simulink model "Chart"  (R2022a)
settings: Solver=FixedStepDiscrete  StartTime=0.0  StopTime=inf  RelTol=1e-3
settings Model: DVExtractedSubsystem=Chart  Creator=attit  LastModifiedBy=attit
settings DebuggingCC: FrameProcessingCompatibilityMsg=none
settings RTWCC: TLCOptions=-aAlwaysIncludeCustomSrc=1
settings ConfigComp: DVMaxProcessTime=4000  DVModelCoverageObjectives=MCDC  DVTestSuiteOptimization=Auto  DVDetectOutOfBounds=on  DVModelReferenceHarness=on  DVHarnessSource=Signal Editor

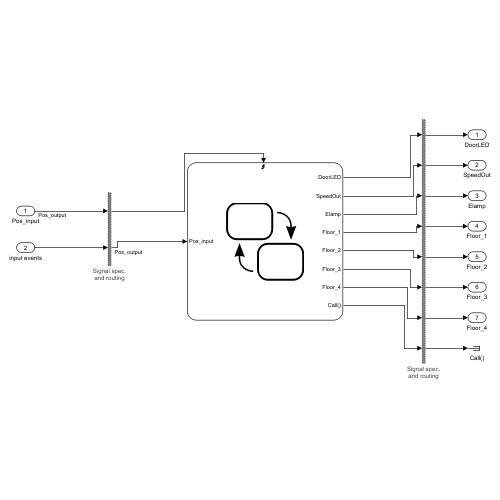
[thumbnail: Simulink's stored preview of the top-level diagram]
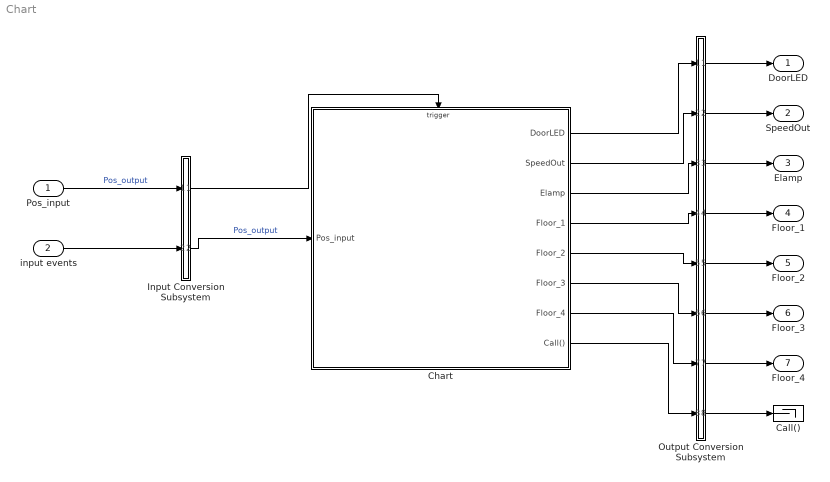
== system Chart ==
  Pos_input : Inport  OutDataTypeStr=double  PortDimensions=[1]  Interpolate=off
  input events : Inport  Port=2  OutDataTypeStr=double  PortDimensions=[7]  Interpolate=off
  Call() : Terminator
  Chart : Stateflow chart  TreatAsAtomicUnit=on
  Input Conversion Subsystem : Subsystem  Tag=__SLT_ICS__  Description=|
      | Signal spec.
      | and routing
      settings: AttributesFormatString=%<Description>
  Output Conversion Subsystem : Subsystem  Tag=__SLT_OCS__  Description=|
      | Signal spec.
      | and routing
      settings: AttributesFormatString=%<Description>
  DoorLED : Outport
  SpeedOut : Outport  Port=2
  Elamp : Outport  Port=3
  Floor_1 : Outport  Port=4
  Floor_2 : Outport  Port=5
  Floor_3 : Outport  Port=6
  Floor_4 : Outport  Port=7
  wires:
  Pos_input/1 -> Input Conversion Subsystem/1(Inport_1)  "Pos_output"
  input events/1 -> Input Conversion Subsystem/2(Inport_2)
  Output Conversion Subsystem/1(Outport_1) -> DoorLED/1
  Output Conversion Subsystem/2(Outport_2) -> SpeedOut/1
  Output Conversion Subsystem/3(Outport_3) -> Elamp/1
  Output Conversion Subsystem/4(Outport_4) -> Floor_1/1
  Output Conversion Subsystem/5(Outport_5) -> Floor_2/1
  Output Conversion Subsystem/6(Outport_6) -> Floor_3/1
  Output Conversion Subsystem/7(Outport_7) -> Floor_4/1
  Output Conversion Subsystem/8(Outport_8) -> Call()/1
  Input Conversion Subsystem/1(Outport_2) -> Chart/Trigger
  Input Conversion Subsystem/2(Outport_1) -> Chart/1(Pos_input)  "Pos_output"
  Chart/1(DoorLED) -> Output Conversion Subsystem/1(Inport_1)
  Chart/2(SpeedOut) -> Output Conversion Subsystem/2(Inport_2)
  Chart/3(Elamp) -> Output Conversion Subsystem/3(Inport_3)
  Chart/4(Floor_1) -> Output Conversion Subsystem/4(Inport_4)
  Chart/5(Floor_2) -> Output Conversion Subsystem/5(Inport_5)
  Chart/6(Floor_3) -> Output Conversion Subsystem/6(Inport_6)
  Chart/7(Floor_4) -> Output Conversion Subsystem/7(Inport_7)
  Chart/8(Call()) -> Output Conversion Subsystem/8(Inport_8)

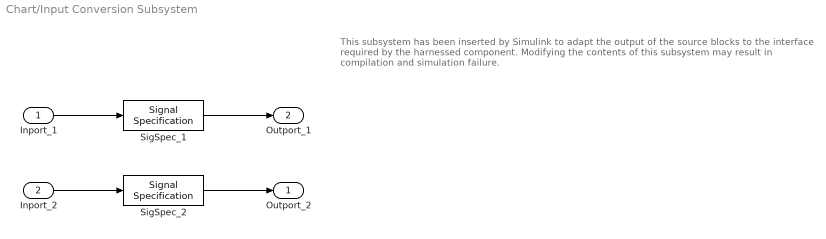
== system Chart/Input Conversion Subsystem ==
  note: This subsystem has been inserted by Simulink to adapt the output of the source blocks to the interface required by the harnessed component.
      |  Modifying the contents of this subsystem may result in compilation and simulation failure.
  Inport_1 : Inport
  Inport_2 : Inport  Port=2
  SigSpec_1 : SignalSpecification  OutDataTypeStr=double  Dimensions=[1]
  SigSpec_2 : SignalSpecification  OutDataTypeStr=double  Dimensions=[7]
  Outport_2 : Outport
  Outport_1 : Outport  Port=2
  wires:
  SigSpec_1/1 -> Outport_1/1
  Inport_1/1 -> SigSpec_1/1
  SigSpec_2/1 -> Outport_2/1
  Inport_2/1 -> SigSpec_2/1

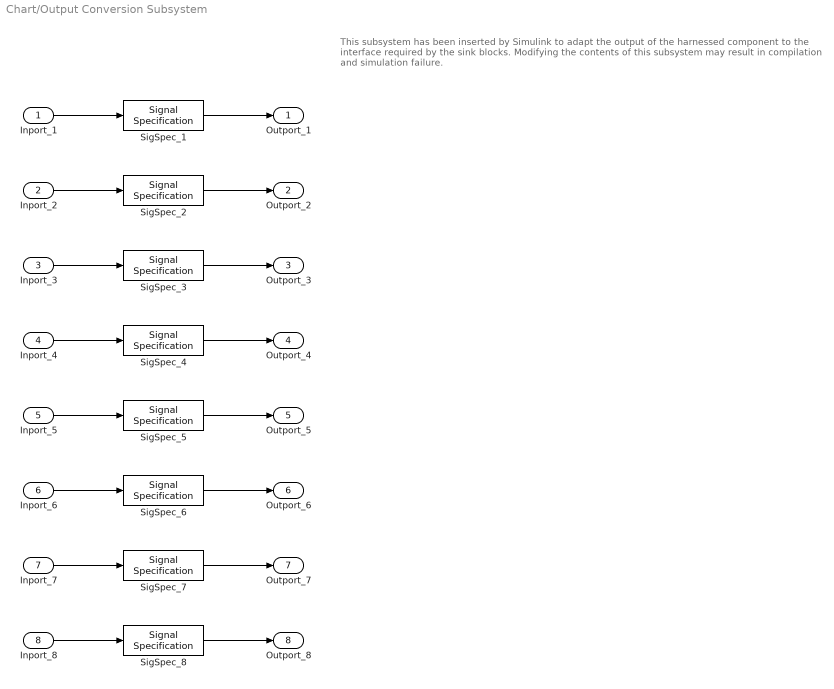
== system Chart/Output Conversion Subsystem ==
  note: This subsystem has been inserted by Simulink to adapt the output of the harnessed component to the interface required by the sink blocks.
      |  Modifying the contents of this subsystem may result in compilation and simulation failure.
  Inport_1 : Inport
  Inport_2 : Inport  Port=2
  Inport_3 : Inport  Port=3
  Inport_4 : Inport  Port=4
  Inport_5 : Inport  Port=5
  Inport_6 : Inport  Port=6
  Inport_7 : Inport  Port=7
  Inport_8 : Inport  Port=8
  SigSpec_{1..7} (7 alike) : SignalSpecification  OutDataTypeStr=double  Dimensions=[1]
  SigSpec_8 : SignalSpecification
  Outport_1 : Outport
  Outport_2 : Outport  Port=2
  Outport_3 : Outport  Port=3
  Outport_4 : Outport  Port=4
  Outport_5 : Outport  Port=5
  Outport_6 : Outport  Port=6
  Outport_7 : Outport  Port=7
  Outport_8 : Outport  Port=8
  wires:
  Inport_1/1 -> SigSpec_1/1
  SigSpec_1/1 -> Outport_1/1
  Inport_2/1 -> SigSpec_2/1
  SigSpec_2/1 -> Outport_2/1
  Inport_3/1 -> SigSpec_3/1
  SigSpec_3/1 -> Outport_3/1
  Inport_4/1 -> SigSpec_4/1
  SigSpec_4/1 -> Outport_4/1
  Inport_5/1 -> SigSpec_5/1
  SigSpec_5/1 -> Outport_5/1
  Inport_6/1 -> SigSpec_6/1
  SigSpec_6/1 -> Outport_6/1
  Inport_7/1 -> SigSpec_7/1
  SigSpec_7/1 -> Outport_7/1
  Inport_8/1 -> SigSpec_8/1
  SigSpec_8/1 -> Outport_8/1

== stateflow chart Chart/Chart ==
  state ElevatorUnitControl [parallel]
    settings: executionOrder=4
    state GO_DOWN
      entry:
      SpeedOut=-0.2
    state OFF
      entry:SpeedOut=0;
      Elamp=0;
    state GO_UP
      entry:SpeedOut=0.2
    state HALT
      entry:SpeedOut=0;
      Elamp=1
    (default) -> OFF
    OFF -> (junction 166) [order 1] : [in(LiftAlgorithm.MOTOR_ON)]
    (junction 166) -> GO_DOWN [order 1] : [Direction<Pos_input]
    GO_DOWN -> (junction 182) [order 1] : [Emergency]
    (junction 166) -> (junction 177) [order 2] : [Direction>Pos_input]
    (junction 182) -> (junction 183)
    GO_DOWN -> OFF [order 2] : [~in(LiftAlgorithm.MOTOR_ON)]
    GO_UP -> OFF [order 2] : [~in(LiftAlgorithm.MOTOR_ON)]
    HALT -> OFF : [Start]
    OFF -> HALT [order 2] : [Emergency]
    (junction 177) -> GO_UP
    GO_UP -> (junction 183) [order 1] : [Emergency]
    (junction 183) -> (junction 184)
    (junction 184) -> HALT
  state RequestServiced(pos) [function]
    note: Do not put any code along
        | the transitions that run
        | down the right side!
    (default) -> (junction 121)
    (junction 121) -> (junction 116) [order 1] : [pos == 1]
    (junction 121) -> (junction 131) [order 2]
    (junction 116) -> (junction 137) : {F1_press=0;}
    (junction 137) -> (junction 120)
    (junction 120) -> (junction 117)
    (junction 131) -> (junction 113) [order 1] : [pos == 2]
    (junction 131) -> (junction 123) [order 2]
    (junction 113) -> (junction 135) : {F2_press=0;}
    (junction 135) -> (junction 117)
    (junction 117) -> (junction 114)
    (junction 123) -> (junction 136) [order 1] : [pos == 3]
    (junction 123) -> (junction 122) [order 2]
    (junction 136) -> (junction 118) : {F3_press=0;}
    (junction 118) -> (junction 114)
    (junction 114) -> (junction 124)
    (junction 122) -> (junction 119) [order 1] : [pos == 4]
    (junction 122) -> (junction 125) [order 2]
    (junction 119) -> (junction 115) : {F4_press=0;}
    (junction 115) -> (junction 124)
    (junction 124) -> (junction 127)
    (junction 127) -> (junction 125)
    (junction 125) -> (junction 129)
  state ret =ValidFloor(indx) [function]
    (default) -> (junction 104)
    (junction 104) -> (junction 110) [order 1] : [abs(indx-1.0)<0.1||abs(indx-2.0)<0.1||abs(indx-3.0)<0.1||abs(indx-4.0)<0.1]
    (junction 110) -> (junction 106) : {ret=1}
    (junction 104) -> (junction 106) [order 2] : {ret=0}
    (junction 106) -> (junction 103)
  state Add(Floor) [function]
    (default) -> (junction 29) : {PressCount=PressCount+1;}
    (junction 29) -> (junction 31) : {Queue(PressCount)=Floor}
  state FloorRequestProcess [parallel]
    settings: executionOrder=1
    state RequestWait
    RequestWait -> RequestWait [order 1] : [F1_evt&&Floor_1~=1]{Add(1);Floor_1=1}
    RequestWait -> RequestWait [order 4] : [F4_evt&&Floor_4~=1]{Add(4);Floor_4=1}
    RequestWait -> RequestWait [order 3] : [F3_evt&&Floor_3~=1]{Add(3);Floor_3=1}
    RequestWait -> RequestWait [order 2] : [F2_evt&&Floor_2~=1]{Add(2);Floor_2=1}
  state Trigger [parallel]
    settings: executionOrder=2
    state TriggerNextchart
    (default) -> TriggerNextchart
    TriggerNextchart -> TriggerNextchart : {Call}
  note: LIFT_ALGORITHM
  state LiftAlgorithm [parallel]
    settings: executionOrder=3
    state DOOR_WAIT
      entry:DoorLED=1;
      RequestServiced(round(Pos_input));
    state DOOR_DONE
      entry:DoorLED=0;
    state WAIT
    state REQUEST_ACCEPTED
    state MOTOR_ON
    state REQUESTED_FLOOR_FOUND
      entry:PressCount=PressCount-1;
      Queue=[Queue(Queue~=round(Pos_input)) zeros(1,length(Queue)-length(Queue(Queue~=round(Pos_input))))];
    (junction 76) -> (junction 75)
    (junction 82) -> (junction 76)
    (default) -> WAIT : {Floor_1=0;Floor_2=0;Floor_3=0;Floor_4=0; Queue=[0 0 0 0]; PressCount=0;}
    (junction 75) -> WAIT
    DOOR_DONE -> (junction 82) [order 2] : [Direction==0]
    DOOR_WAIT -> DOOR_DONE : [after(5,sec)]
    WAIT -> REQUEST_ACCEPTED : [PressCount>0]{Direction=Queue(1)}
    REQUEST_ACCEPTED -> DOOR_WAIT [order 2] : [Direction==Pos_input]{Direction=0;Queue=[Queue(Queue~=round(Pos_input)) zeros(1,length(Queue)-length(Queue(Queue~=round(Pos_input))))];}
    REQUESTED_FLOOR_FOUND -> DOOR_WAIT [order 2]
    REQUESTED_FLOOR_FOUND -> DOOR_WAIT [order 1] : [abs(Direction-Pos_input)<0.1]{Direction=0;}
    DOOR_DONE -> (junction 78) [order 1] : [Direction~=0]
    REQUEST_ACCEPTED -> MOTOR_ON [order 1] : [Direction~=Pos_input]
    (junction 79) -> MOTOR_ON
    MOTOR_ON -> REQUESTED_FLOOR_FOUND : [1==ValidFloor(Pos_input)&&1==any(Queue(:)==round(Pos_input))]
    (junction 78) -> (junction 79)
  note: ElevatorUnitControl
  (default) -> RequestWait : {Floor_1=0;Floor_2=0;Floor_3=0;Floor_4=0; Queue=[0 0 0 0]; PressCount=0;}
  data: pos function_input; indx function_input; ret function_output; Floor function_input; Queue local size=[1 4]; Pos_input input [1..4]; DoorLED output; PressCount local; Direction local; SpeedOut output; Elamp output; Floor_1 output; Floor_2 output; Floor_3 output; Floor_4 output
  events: Trigger input RISING_EDGE_EVENT; Call output FUNCTION_CALL_EVENT; F1_evt input RISING_EDGE_EVENT; F2_evt input RISING_EDGE_EVENT; F3_evt input RISING_EDGE_EVENT; F4_evt input RISING_EDGE_EVENT; Start input RISING_EDGE_EVENT; Emergency input RISING_EDGE_EVENT
